simulink model "AHRS_Voter"  (R2023b)
settings: configuration reference "csSingleInstance" (kept outside this file)
libraries: simulink x1
Description:
  | This model implements the AHRS voting algorithm of the helicopter flight control software.
settings Model: DataDictionary=DD_AHRS_Voter.sldd  EnableAccessToBaseWorkspace=off  Creator=The MathWorks, Inc.  LastModifiedBy=The MathWorks, Inc.
settings ConfigSetRef: SourceName=csSingleInstance

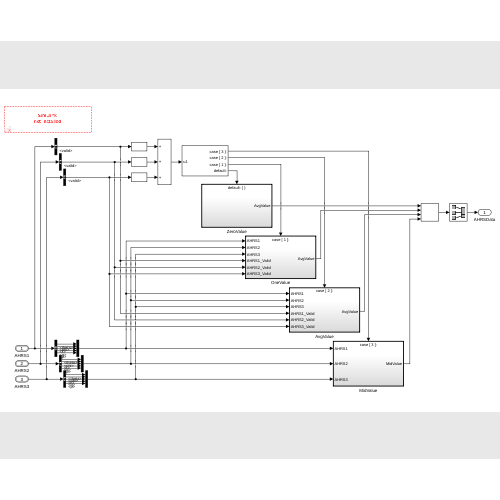
[thumbnail: Simulink's stored preview of the top-level diagram]
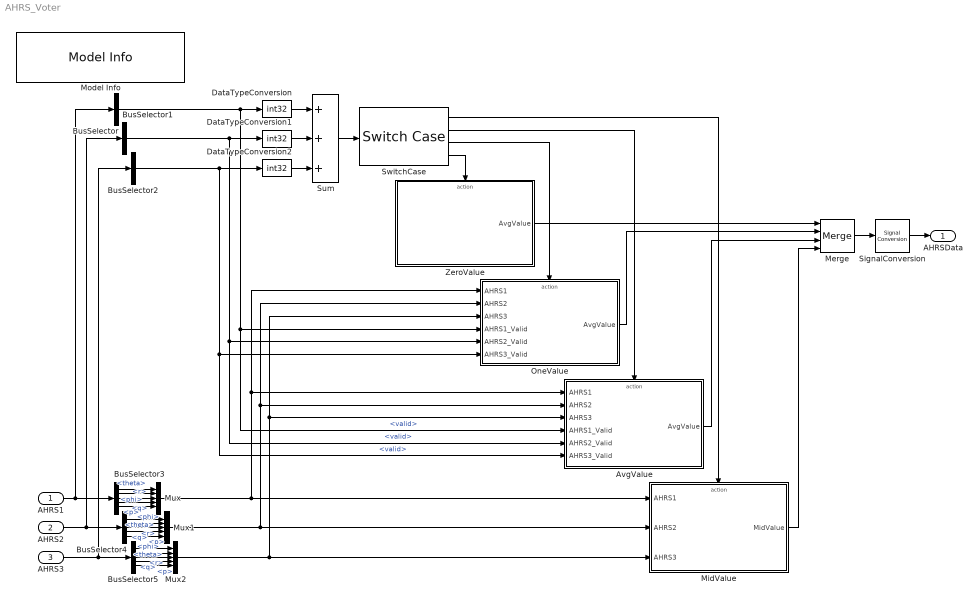
== system AHRS_Voter ==
  AHRS1 : Inport  OutDataTypeStr=Bus: AHRS_Bus  PortDimensions=1  SampleTime=0.01  BusOutputAsStruct=on
  AHRS2 : Inport  Port=2  OutDataTypeStr=Bus: AHRS_Bus  PortDimensions=1  SampleTime=0.01  BusOutputAsStruct=on
  AHRS3 : Inport  Port=3  OutDataTypeStr=Bus: AHRS_Bus  PortDimensions=1  SampleTime=0.01  BusOutputAsStruct=on
  AvgValue : Subsystem  TreatAsAtomicUnit=on
      settings: RTWSystemCode=Inline
  BusSelector : BusSelector  OutputSignals=valid
  BusSelector1 : BusSelector  OutputSignals=valid
  BusSelector2 : BusSelector  OutputSignals=valid
  BusSelector3 : BusSelector  OutputSignals=theta,phi,r,q,p
  BusSelector4 : BusSelector  OutputSignals=theta,phi,r,q,p
  BusSelector5 : BusSelector  OutputSignals=theta,phi,r,q,p
  DataTypeConversion : DataTypeConversion  OutDataTypeStr=int32  SaturateOnIntegerOverflow=off  RndMeth=Floor
  DataTypeConversion1 : DataTypeConversion  OutDataTypeStr=int32  SaturateOnIntegerOverflow=off  RndMeth=Floor
  DataTypeConversion2 : DataTypeConversion  OutDataTypeStr=int32  SaturateOnIntegerOverflow=off  RndMeth=Floor
  Merge : Merge  Inputs=4
  MidValue : Subsystem  TreatAsAtomicUnit=on
      settings: RTWSystemCode=Inline
  Model Info : simulink/Model-Wide Utilities/Model Info  Frame=on  DisplayStringWithTags=|  HorizontalTextAlignment=Center  LeftAlignmentValue=0.5
      | Model Name: %<ModelName>
      | Model Version: %<ModelVersion>
      | Last Modified: %<LastModificationDate>
  Mux : Mux  Inputs=5
  Mux1 : Mux  Inputs=5
  Mux2 : Mux  Inputs=5
  OneValue : Subsystem  TreatAsAtomicUnit=on
      settings: RTWSystemCode=Inline
  SignalConversion : SignalConversion  OverrideOpt=on
  Sum : Sum  Inputs=+++  OutDataTypeStr=int32
  SwitchCase : SwitchCase  CaseConditions={3, 2, 1}
  ZeroValue : Subsystem  TreatAsAtomicUnit=on
      settings: RTWSystemCode=Inline
  AHRSData : Outport  VectorParamsAs1DForOutWhenUnconnected=off
  wires:
  Sum/1 -> SwitchCase/1
  AHRS1/1 -> BusSelector/1, BusSelector3/1
  AHRS2/1 -> BusSelector4/1, BusSelector1/1
  AHRS3/1 -> BusSelector5/1, BusSelector2/1
  BusSelector/1 -> DataTypeConversion/1, AvgValue/4(AHRS1_Valid), OneValue/4(AHRS1_Valid)  "<valid>"
  BusSelector1/1 -> DataTypeConversion1/1, AvgValue/5(AHRS2_Valid), OneValue/5(AHRS2_Valid)  "<valid>"
  BusSelector2/1 -> DataTypeConversion2/1, AvgValue/6(AHRS3_Valid), OneValue/6(AHRS3_Valid)  "<valid>"
  Mux/1 -> OneValue/1(AHRS1), AvgValue/1(AHRS1), MidValue/1(AHRS1)
  BusSelector3/1 -> Mux/1  "<theta>"
  BusSelector3/2 -> Mux/2  "<phi>"
  BusSelector3/3 -> Mux/3  "<r>"
  BusSelector3/4 -> Mux/4  "<q>"
  BusSelector3/5 -> Mux/5  "<p>"
  BusSelector4/1 -> Mux1/1  "<theta>"
  BusSelector4/2 -> Mux1/2  "<phi>"
  BusSelector4/3 -> Mux1/3  "<r>"
  BusSelector4/4 -> Mux1/4  "<q>"
  BusSelector4/5 -> Mux1/5  "<p>"
  BusSelector5/1 -> Mux2/1  "<theta>"
  BusSelector5/2 -> Mux2/2  "<phi>"
  BusSelector5/3 -> Mux2/3  "<r>"
  BusSelector5/4 -> Mux2/4  "<q>"
  BusSelector5/5 -> Mux2/5  "<p>"
  Mux1/1 -> AvgValue/2(AHRS2), OneValue/2(AHRS2), MidValue/2(AHRS2)
  Mux2/1 -> AvgValue/3(AHRS3), OneValue/3(AHRS3), MidValue/3(AHRS3)
  SwitchCase/4 -> ZeroValue/Action
  SwitchCase/3 -> OneValue/Action
  SwitchCase/2 -> AvgValue/Action
  SwitchCase/1 -> MidValue/Action
  Merge/1 -> SignalConversion/1
  ZeroValue/1(AvgValue) -> Merge/1
  OneValue/1(AvgValue) -> Merge/2
  AvgValue/1(AvgValue) -> Merge/3
  MidValue/1(MidValue) -> Merge/4
  DataTypeConversion/1 -> Sum/1
  DataTypeConversion1/1 -> Sum/2
  DataTypeConversion2/1 -> Sum/3
  SignalConversion/1 -> AHRSData/1

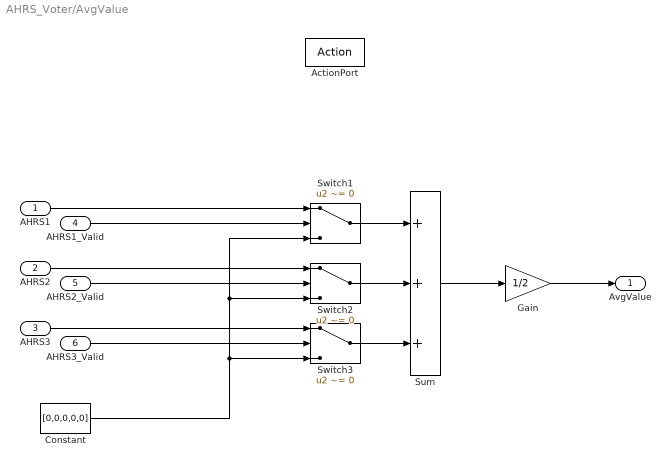
== system AHRS_Voter/AvgValue ==
  AHRS1 : Inport
  AHRS2 : Inport  Port=2
  AHRS3 : Inport  Port=3
  AHRS1_Valid : Inport  Port=4  OutDataTypeStr=boolean  PortDimensions=1
  AHRS2_Valid : Inport  Port=5  OutDataTypeStr=boolean  PortDimensions=1
  AHRS3_Valid : Inport  Port=6  OutDataTypeStr=boolean  PortDimensions=1
  ActionPort : ActionPort  ActionPortLabel=case [ 2 ]:
  Constant : Constant  Value=[0,0,0,0,0]
  Gain : Gain  Gain=1/2
  Sum : Sum  Inputs=+++
  Switch1 : Switch  Criteria=u2 ~= 0  SaturateOnIntegerOverflow=off  InputSameDT=off
  Switch2 : Switch  Criteria=u2 ~= 0  SaturateOnIntegerOverflow=off  InputSameDT=off
  Switch3 : Switch  Criteria=u2 ~= 0  SaturateOnIntegerOverflow=off  InputSameDT=off
  AvgValue : Outport  VectorParamsAs1DForOutWhenUnconnected=off
  wires:
  AHRS3/1 -> Switch3/1
  AHRS2/1 -> Switch2/1
  AHRS3_Valid/1 -> Switch3/2
  AHRS2_Valid/1 -> Switch2/2
  Switch3/1 -> Sum/3
  Switch2/1 -> Sum/2
  Switch1/1 -> Sum/1
  AHRS1/1 -> Switch1/1
  AHRS1_Valid/1 -> Switch1/2
  Sum/1 -> Gain/1
  Gain/1 -> AvgValue/1
  Constant/1 -> Switch3/3, Switch2/3, Switch1/3

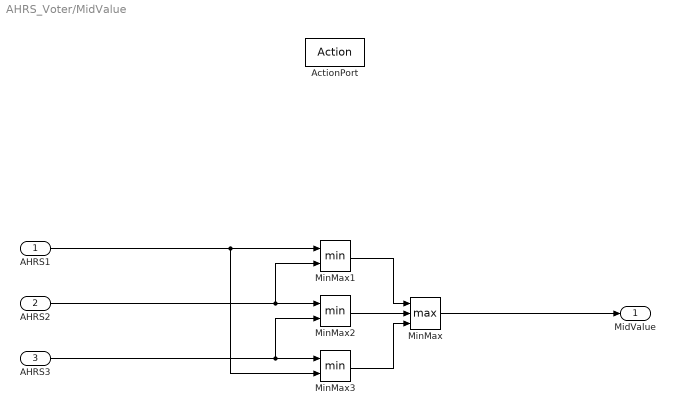
== system AHRS_Voter/MidValue ==
  AHRS1 : Inport
  AHRS2 : Inport  Port=2
  AHRS3 : Inport  Port=3
  ActionPort : ActionPort  ActionPortLabel=case [ 3 ]:
  MinMax : MinMax  Function=max  Inputs=3
  MinMax1 : MinMax  Inputs=2
  MinMax2 : MinMax  Inputs=2
  MinMax3 : MinMax  Inputs=2
  MidValue : Outport  VectorParamsAs1DForOutWhenUnconnected=off
  wires:
  MinMax/1 -> MidValue/1
  MinMax2/1 -> MinMax/2
  AHRS2/1 -> MinMax2/1, MinMax1/2
  AHRS3/1 -> MinMax3/1, MinMax2/2
  AHRS1/1 -> MinMax1/1, MinMax3/2
  MinMax1/1 -> MinMax/1
  MinMax3/1 -> MinMax/3

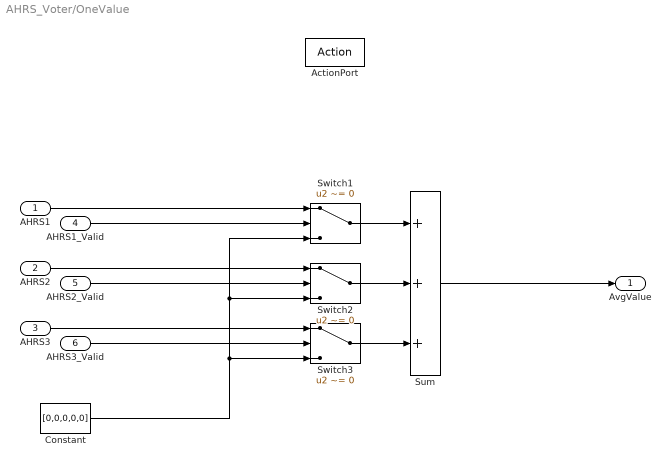
== system AHRS_Voter/OneValue ==
  AHRS1 : Inport
  AHRS2 : Inport  Port=2
  AHRS3 : Inport  Port=3
  AHRS1_Valid : Inport  Port=4  OutDataTypeStr=boolean  PortDimensions=1
  AHRS2_Valid : Inport  Port=5  OutDataTypeStr=boolean  PortDimensions=1
  AHRS3_Valid : Inport  Port=6  OutDataTypeStr=boolean  PortDimensions=1
  ActionPort : ActionPort  ActionPortLabel=case [ 1 ]:
  Constant : Constant  Value=[0,0,0,0,0]
  Sum : Sum  Inputs=+++
  Switch1 : Switch  Criteria=u2 ~= 0  SaturateOnIntegerOverflow=off  InputSameDT=off
  Switch2 : Switch  Criteria=u2 ~= 0  SaturateOnIntegerOverflow=off  InputSameDT=off
  Switch3 : Switch  Criteria=u2 ~= 0  SaturateOnIntegerOverflow=off  InputSameDT=off
  AvgValue : Outport  VectorParamsAs1DForOutWhenUnconnected=off
  wires:
  Constant/1 -> Switch1/3, Switch2/3, Switch3/3
  Sum/1 -> AvgValue/1
  AHRS1_Valid/1 -> Switch1/2
  AHRS1/1 -> Switch1/1
  Switch1/1 -> Sum/1
  Switch2/1 -> Sum/2
  Switch3/1 -> Sum/3
  AHRS2_Valid/1 -> Switch2/2
  AHRS3_Valid/1 -> Switch3/2
  AHRS2/1 -> Switch2/1
  AHRS3/1 -> Switch3/1

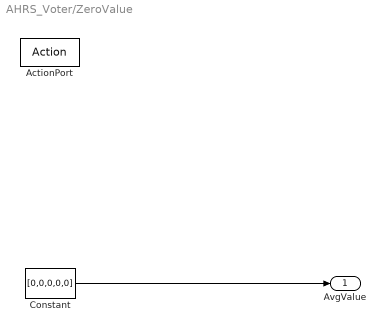
== system AHRS_Voter/ZeroValue ==
  ActionPort : ActionPort  ActionPortLabel=default:
  Constant : Constant  Value=[0,0,0,0,0]  SampleTime=-1
  AvgValue : Outport  VectorParamsAs1DForOutWhenUnconnected=off
  wires:
  Constant/1 -> AvgValue/1
